simulink model "UsingArrayC"  (R2017a)
settings: Solver=FixedStepAuto  StartTime=0.0  StopTime=10.0  FixedStep=0.1  RelTol=1e-3
settings Model: Creator=TSu  LastModifiedBy=TSu
settings SolverCC: AutoInsertRateTranBlk=on

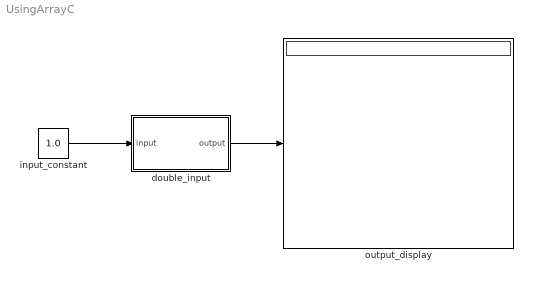
== system UsingArrayC ==
  double_input : MATLAB Function  TreatAsAtomicUnit=on
  input_constant : Constant  Value=1.0
  output_display : Display
  wires:
  input_constant/1 -> double_input/1(input)
  double_input/1(output) -> output_display/1

== matlab function UsingArrayC/double_input ==
  data: input input; output output
function output = double_input(input)
% double_input: This MATLAB function outputs the double of the input
% variable.

% output = 2.0 * input;

% output = 0.0;
% output = coder.ceval('myMult2', input);

% output = 0.0
% input_copy = input;
% coder.ceval('myMult2', coder.wref(input_copy));
% output = input_copy;

output = zeros(10,3);
tempt = zeros(10,3);
[num_rows,num_cols] = size(tempt);
coder.ceval('update_array', coder.wref(tempt), int32(num_rows), int32(num_cols));
output = tempt;

% Specify the locations of myMult2.h and myMult2.c
coder.extrinsic('pwd', 'fullfile');
customDir = coder.const(fullfile(pwd, 'c_codes'));
coder.updateBuildInfo('addIncludePaths', customDir);
coder.updateBuildInfo('addSourcePaths', customDir);
coder.cinclude('myMult2.h'); % includes a header file in generated C/C++ source code.
coder.updateBuildInfo('addSourceFiles', 'myMult2.c');
end
